simulink model "ackerman_ROS_controller_neuronal"  (R2024a)
settings: Solver=FixedStepDiscrete  StartTime=0.0  StopTime=70  FixedStep=0.1  RelTol=1e-3
undefined symbols (not defined in the file or in its folder): Angular, Linear
libraries: neural x47, robotlib x15, robotcorelib x1
(part 2 of 2)

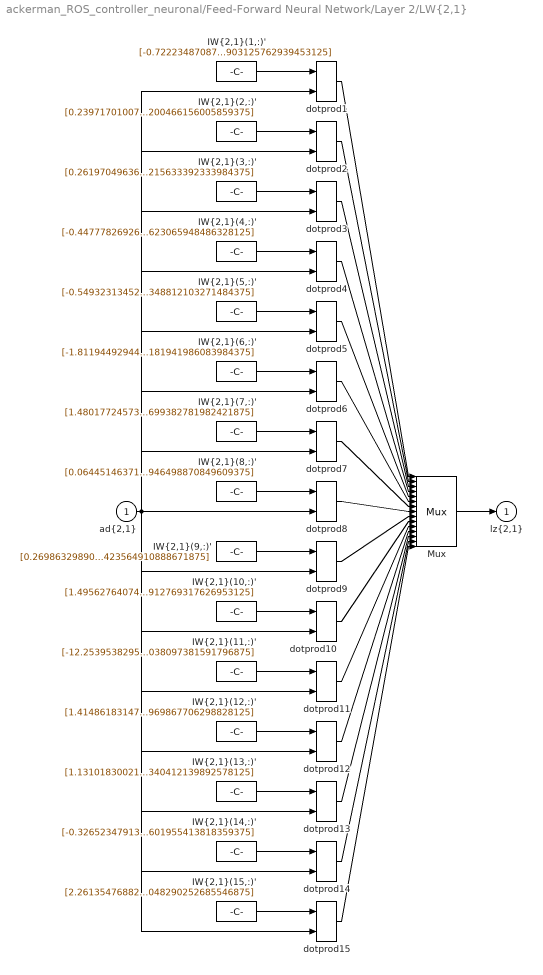
== system ackerman_ROS_controller_neuronal/Feed-Forward Neural Network/Layer 2/LW{2,1} ==
  "ad{2,1}" : Inport  PortDimensions=25  SampleTime=0.1
      mask Display: e = 0.06;c1 = [120 230 180]/255;c2 = ([120 230 180]+0)/(256+128);c3 = ([120 230 180]+128)/(256+128);patch([0 1 1 0],[0 0 1 1],c1);patch([0 1 1 1-e 1-e 0+e],[0 0 1 1-e 0+e 0+e],c2);patch([0 0 1 1-e 0+e 0+e],[0 1 1 1-e 1-e 0+e],c3);plot([0 1 1 0 0],[0 0 1 1 0]);
  "IW{2,1}(1,:)'" : Constant  Value=[-0.7222348708729093846869773187790997326374053955078125;0.0981793588010296536250365306841558776795864105224609375;0.1371759683882359526219119061352103017270565032958984375;0.0730258607750217392240443814444006420671939849853515625;-1.372802742190014857470714559894986450672149658203125;-1.8212743748848574387722010214929468929767608642578125;-1.5267678279169134558657106026657857000827789306640625;1.4479084045406518388432459687464870512485504150390625;-0.13063321599715915777295549560221843421459197998046875;1.712382502643198467495722070452757179737091064453125;-0.1827473613784254269365447953532566316425800323486328125;-1.0574757090524122826735720082069747149944305419921875;-1.0665010937239696175993231008760631084442138671875;-0.9024666040768736241517444796045310795307159423828125;-1.8865157325392905018901501534855924546718597412109375;1.318039630886072899329519714228808879852294921875;1.1464077279038644707753746843081898987293243408203125;-0.97169709672360526919732137685059569776058197021484375;-2.487878129250618020051888379384763538837432861328125;-0.9738457646549019131043678498826920986175537109375;0.34793062286432674401481790482648648321628570556640625;0.01100840170375953601389351632633406552486121654510498046875;1.6560578546683313305720730568282306194305419921875;-2.101274677924584555199771784828044474124908447265625;2.983503581776024038418881900724954903125762939453125]
      mask Display: e = 0.06;c1 = [120 150 230]/255;c2 = ([120 150 230]+0)/383;c3 = ([120 150 230]+128)/383;patch([0 1 1 0],[0 0 1 1],c1);patch([0 1 1 1-e 1-e 0+e],[0 0 1 1-e 0+e 0+e],c2);patch([0 0 1 1-e 0+e 0+e],[0 1 1 1-e 1-e 0+e],c3);plot([0 1 1 0 0],[0 0 1 1 0]);disp('weights');
  "IW{2,1}(10,:)'" : Constant  Value=[1.4956276407477755441277622594498097896575927734375;-0.788962805301818281833448054385371506214141845703125;0.269669087111882144203178768293582834303379058837890625;-0.292657048209959469442509316650102846324443817138671875;-2.133692028425654196865934864035807549953460693359375;-0.39117674700785476371578397447592578828334808349609375;0.581263930568486131278405082412064075469970703125;0.97155478441386866617079931529588066041469573974609375;-2.073983957749963025207762257196009159088134765625;2.731327761950456789463714812882244586944580078125;-0.4915888766656066888316445329110138118267059326171875;-2.3179880946341011593858638661913573741912841796875;0.09301131783168821443030793716388870961964130401611328125;0.1436793922233029208168630930231302045285701751708984375;-1.64205595454593389348474374855868518352508544921875;0.2132037752463056268226182510261423885822296142578125;0.27785129634182259561470118569559417665004730224609375;1.5674675258729935389823140212683938443660736083984375;-0.8311551921900461881165256272652186453342437744140625;-1.7108512116470517838706655311398208141326904296875;0.07415612580187225244543469671043567359447479248046875;-0.55140252940727052521907580739934928715229034423828125;-1.38513208025195666550644091330468654632568359375;0.1518428514926022654396575717328232713043689727783203125;2.596690078219698438743989754584617912769317626953125]
      mask Display: e = 0.06;c1 = [120 150 230]/255;c2 = ([120 150 230]+0)/383;c3 = ([120 150 230]+128)/383;patch([0 1 1 0],[0 0 1 1],c1);patch([0 1 1 1-e 1-e 0+e],[0 0 1 1-e 0+e 0+e],c2);patch([0 0 1 1-e 0+e 0+e],[0 1 1 1-e 1-e 0+e],c3);plot([0 1 1 0 0],[0 0 1 1 0]);disp('weights');
  "IW{2,1}(11,:)'" : Constant  Value=[-12.253953829568370537117516505531966686248779296875;4.39303208527887623091601199121214449405670166015625;0.38223307212810386790380334787187166512012481689453125;-1.9037658357750879556391510050161741673946380615234375;-0.95260750474161459688815511981374584138393402099609375;5.360034857704107480458333157002925872802734375;6.67310871356777823848460684530436992645263671875;2.729141390269420153202872825204394757747650146484375;-1.915432689159779489074253433500416576862335205078125;-1.018409021534567582278896225034259259700775146484375;0.3096668608063126715279622658272273838520050048828125;-0.356772271992063794154859124319045804440975189208984375;-3.5098980230815488567941429209895431995391845703125;-2.42911505781934788927856061491183936595916748046875;-3.80273708191338233319811479304917156696319580078125;2.49722685927970733388292501331306993961334228515625;-0.8878414190837864428118564319447614252567291259765625;2.402914930610447807879381798557005822658538818359375;-0.5057975403114471912857652569073252379894256591796875;7.45380146518667441313255039858631789684295654296875;1.7300526442494590373399887539562769234180450439453125;2.665766658331240268609008126077242195606231689453125;1.8102918202158633231846351918647997081279754638671875;-0.98601708086775996520145781687460839748382568359375;1.442751514700642445632183807902038097381591796875]
      mask Display: e = 0.06;c1 = [120 150 230]/255;c2 = ([120 150 230]+0)/383;c3 = ([120 150 230]+128)/383;patch([0 1 1 0],[0 0 1 1],c1);patch([0 1 1 1-e 1-e 0+e],[0 0 1 1-e 0+e 0+e],c2);patch([0 0 1 1-e 0+e 0+e],[0 1 1 1-e 1-e 0+e],c3);plot([0 1 1 0 0],[0 0 1 1 0]);disp('weights');
  "IW{2,1}(12,:)'" : Constant  Value=[1.414861831478989362409492969163693487644195556640625;1.2707933400524071831938499599345959722995758056640625;1.34394123583657698617344067315571010112762451171875;1.5462306076190726056296398382983170449733734130859375;-5.17509624264692735806647760909982025623321533203125;2.824180089653766767554543548612855374813079833984375;-1.82988593402526600328883432666771113872528076171875;-3.2592273475407065319586763507686555385589599609375;-1.928758399229578923694816694478504359722137451171875;-1.34087555628182286682203994132578372955322265625;-5.07940803163818177523580743581987917423248291015625;1.5511947868706601472155170995392836630344390869140625;-2.096771476592278471429153796634636819362640380859375;0.90357692537882805527971186165814287960529327392578125;-1.337567839827941806873923269449733197689056396484375;-0.79672981490855487862745576421730220317840576171875;-0.4541749841010995769607916372478939592838287353515625;2.14134792906865190076359795057214796543121337890625;-3.362985062282791037802098799147643148899078369140625;-1.466686761802152627609530100016854703426361083984375;-4.816526752401596667141348007135093212127685546875;1.9420442507405712984080992100643925368785858154296875;0.1615625324561887066199261653309804387390613555908203125;-0.04622279232351557409774756024489761330187320709228515625;3.825540516566335202952586769242770969867706298828125]
      mask Display: e = 0.06;c1 = [120 150 230]/255;c2 = ([120 150 230]+0)/383;c3 = ([120 150 230]+128)/383;patch([0 1 1 0],[0 0 1 1],c1);patch([0 1 1 1-e 1-e 0+e],[0 0 1 1-e 0+e 0+e],c2);patch([0 0 1 1-e 0+e 0+e],[0 1 1 1-e 1-e 0+e],c3);plot([0 1 1 0 0],[0 0 1 1 0]);disp('weights');
  "IW{2,1}(13,:)'" : Constant  Value=[1.131018300215737237834900952293537557125091552734375;4.6569848027918627764165648841299116611480712890625;0.2344222257143036836080085549838258884847164154052734375;-1.9242483801722425340585687081329524517059326171875;0.63069029440676704911794558938709087669849395751953125;-0.64797978029724834225788754338282160460948944091796875;1.5346118234120551537813526010722853243350982666015625;-3.07598490301061300300489165238104760646820068359375;-1.0483748074715124598554893964319489896297454833984375;4.582483484907502457872396917082369327545166015625;-0.775742089778314269921111190342344343662261962890625;2.773228499954765169377424172125756740570068359375;-2.9959296210777655034007693757303059101104736328125;-0.93210670025544517525162291349261067807674407958984375;0.57584394096119317918436308900709263980388641357421875;1.672267185378192966282995257643051445484161376953125;1.4951734432408445574225197560735978186130523681640625;-1.1348966277614584985400369987473823130130767822265625;1.0463170313689882373608952548238448798656463623046875;-2.95346669820664242678276423248462378978729248046875;1.6040671880945283067632090023835189640522003173828125;1.7640246337201224147150924181914888322353363037109375;-2.450281737022660166758214472793042659759521484375;0.81620673218923356362353160875500179827213287353515625;-0.003525358734461532528303706612859969027340412139892578125]
      mask Display: e = 0.06;c1 = [120 150 230]/255;c2 = ([120 150 230]+0)/383;c3 = ([120 150 230]+128)/383;patch([0 1 1 0],[0 0 1 1],c1);patch([0 1 1 1-e 1-e 0+e],[0 0 1 1-e 0+e 0+e],c2);patch([0 0 1 1-e 0+e 0+e],[0 1 1 1-e 1-e 0+e],c3);plot([0 1 1 0 0],[0 0 1 1 0]);disp('weights');
  "IW{2,1}(14,:)'" : Constant  Value=[-0.3265234791349171938890094679663889110088348388671875;-1.1396787488998636472814496300998143851757049560546875;0.659566474006498371096540722646750509738922119140625;0.272697770417793972086428766488097608089447021484375;-5.0464894937421629350637886091135442256927490234375;-0.460730509190456605228547459773835726082324981689453125;0.347248761171756681331856952965608797967433929443359375;-1.8789288689546033150890025353874079883098602294921875;-2.372149876109781896360573227866552770137786865234375;-1.47061283460651903709504040307365357875823974609375;0.304297002840665686829169089833158068358898162841796875;0.45927046314568908957909343371284194290637969970703125;0.00965151118650432564283203618060724693350493907928466796875;-0.0089597391306133720989546276314285933040082454681396484375;1.4480728283000530165480768118868581950664520263671875;-0.259619475803844868000425094578531570732593536376953125;-3.23881172172160081146330412593670189380645751953125;1.4267256202362077477374668887932784855365753173828125;0.041194781003231463467617601281745010055601596832275390625;-0.0296330333925509982473389669621610664762556552886962890625;0.143119096384909549879438372954609803855419158935546875;2.041884735769875280908536296919919550418853759765625;-1.60335254904017698862617180566303431987762451171875;0.73699941051827277949115568844717927277088165283203125;0.77850010350764475841600642525008879601955413818359375]
      mask Display: e = 0.06;c1 = [120 150 230]/255;c2 = ([120 150 230]+0)/383;c3 = ([120 150 230]+128)/383;patch([0 1 1 0],[0 0 1 1],c1);patch([0 1 1 1-e 1-e 0+e],[0 0 1 1-e 0+e 0+e],c2);patch([0 0 1 1-e 0+e 0+e],[0 1 1 1-e 1-e 0+e],c3);plot([0 1 1 0 0],[0 0 1 1 0]);disp('weights');
  "IW{2,1}(15,:)'" : Constant  Value=[2.261354768825730499060000511235557496547698974609375;-1.0449084387729128398092370844096876680850982666015625;0.498644497600040315088421039035893045365810394287109375;0.87165995268127527406676335886004380881786346435546875;-0.2117581073043853512327672206083661876618862152099609375;0.589209338323644526980160662787966430187225341796875;0.56663579855300560961239852986182086169719696044921875;-1.712363214106411124504347753827460110187530517578125;-0.21948370763189817278515647558378987014293670654296875;-0.2630627043740132453564228853792883455753326416015625;-0.9383844632776570104937263749889098107814788818359375;0.608847469718369893598719500005245208740234375;-0.84536117835731550140820900196558795869350433349609375;-0.386280090041679902146398717377451248466968536376953125;0.99837546791996378825473357210285030305385589599609375;0.75469207194089904522371625716914422810077667236328125;1.5421940189576950341887595641310326755046844482421875;-1.36341207684782528275491131353192031383514404296875;-0.2430661277789683272221310517124948091804981231689453125;-0.51870593074241233555454755332903005182743072509765625;0.73854121379737935892961786521482281386852264404296875;-1.1794436948531548114971201357548125088214874267578125;0.27331330562690603347419937563245184719562530517578125;-0.3090746830244601728310271937516517937183380126953125;0.6425613674276131614959695070865564048290252685546875]
      mask Display: e = 0.06;c1 = [120 150 230]/255;c2 = ([120 150 230]+0)/383;c3 = ([120 150 230]+128)/383;patch([0 1 1 0],[0 0 1 1],c1);patch([0 1 1 1-e 1-e 0+e],[0 0 1 1-e 0+e 0+e],c2);patch([0 0 1 1-e 0+e 0+e],[0 1 1 1-e 1-e 0+e],c3);plot([0 1 1 0 0],[0 0 1 1 0]);disp('weights');
  "IW{2,1}(2,:)'" : Constant  Value=[0.2397170100764628164480285477111465297639369964599609375;-1.7860235372168258294323095469735562801361083984375;-0.1909341104956231160993951334603480063378810882568359375;1.089794091494230343641902436502277851104736328125;-0.25454316182217018305067313121980987489223480224609375;0.4322605672483723626697837971732951700687408447265625;-0.2048728567615103468568804601090960204601287841796875;1.0010713515385096794574337764061056077480316162109375;0.295535753540752732515528578005614690482616424560546875;1.92087198018925864317907326039858162403106689453125;-1.605335300954486843494350978289730846881866455078125;-0.348238180518220807879714584487373940646648406982421875;-0.213920007137737899771678939941921271383762359619140625;-0.15827597510949320547268825976061634719371795654296875;-1.87095494522964767014627796015702188014984130859375;0.5537583126068204020242546903318725526332855224609375;3.393669821761664540105130072333849966526031494140625;-0.93735669682763977927919540888979099690914154052734375;-0.489971756418236259467136051171110011637210845947265625;-0.52340342207687695630369262289605103433132171630859375;-0.045709986400645892523630919868082855828106403350830078125;-1.6593880364962318996191470432677306234836578369140625;0.298272634381946233350646480175782926380634307861328125;-2.248105500618230667697616809164173901081085205078125;-0.6680062031411961864790782783529721200466156005859375]
      mask Display: e = 0.06;c1 = [120 150 230]/255;c2 = ([120 150 230]+0)/383;c3 = ([120 150 230]+128)/383;patch([0 1 1 0],[0 0 1 1],c1);patch([0 1 1 1-e 1-e 0+e],[0 0 1 1-e 0+e 0+e],c2);patch([0 0 1 1-e 0+e 0+e],[0 1 1 1-e 1-e 0+e],c3);plot([0 1 1 0 0],[0 0 1 1 0]);disp('weights');
  "IW{2,1}(3,:)'" : Constant  Value=[0.261970496368628624761498713269247673451900482177734375;-0.60739888280470599735139103358960710465908050537109375;0.5564599097384554937661960138939321041107177734375;-0.374375860105218893902900845205294899642467498779296875;-0.78299327263608053950605381032801233232021331787109375;0.06357714215609898411596390133126988075673580169677734375;1.4192641090693587369031547495978884398937225341796875;2.51693998010587183244979314622469246387481689453125;5.6294623510423189571838520350866019725799560546875;-1.286464539985229027507784849149174988269805908203125;-0.12354346668453076996119222030756645835936069488525390625;-1.1111505971322819252833369318977929651737213134765625;0.91159341951149153171485295388265512883663177490234375;-0.39232622808146577764176754499203525483608245849609375;0.1402175853463884236393965920797199942171573638916015625;0.56925765277390716345706778156454674899578094482421875;0.92059763213383638547071541324839927256107330322265625;0.94367513594503582563532972926623187959194183349609375;0.10236138442994859032442178659039200283586978912353515625;-4.77041041420481537471687261131592094898223876953125;0.168770138560168536656647120253182947635650634765625;-0.26194322280417259296569909565732814371585845947265625;-0.475774971764924725636802804729086346924304962158203125;-1.5736736682102014928119615433388389647006988525390625;1.431688367580961962488572680740617215633392333984375]
      mask Display: e = 0.06;c1 = [120 150 230]/255;c2 = ([120 150 230]+0)/383;c3 = ([120 150 230]+128)/383;patch([0 1 1 0],[0 0 1 1],c1);patch([0 1 1 1-e 1-e 0+e],[0 0 1 1-e 0+e 0+e],c2);patch([0 0 1 1-e 0+e 0+e],[0 1 1 1-e 1-e 0+e],c3);plot([0 1 1 0 0],[0 0 1 1 0]);disp('weights');
  "IW{2,1}(4,:)'" : Constant  Value=[-0.44777826926594743728315961561747826635837554931640625;-3.383725423316843006205090205185115337371826171875;-0.78746623535786863801178014909964986145496368408203125;2.1890108502724530126215540803968906402587890625;-0.352996033818494481248961847086320631206035614013671875;-3.3560840870066943608662768383510410785675048828125;-0.47181060041684241834758495315327309072017669677734375;0.1349511593528751329795767333052936010062694549560546875;0.19762711076085504036115025883191265165805816650390625;2.0448312559800871923698650789447128772735595703125;0.351244934439365941170052565212245099246501922607421875;-4.7063534150473866901620567659847438335418701171875;-0.467541956344167675130307770814397372305393218994140625;1.149312339418189221618149531423114240169525146484375;-4.802232561185082460042394814081490039825439453125;-0.86280849768037015667943023800035007297992706298828125;-1.79669457532872645089128127438016235828399658203125;1.9719066394604662928458083115401677787303924560546875;-0.409838122969578666499046448734588921070098876953125;-0.198989210572557084777400859820772893726825714111328125;0.07149902547644758354916660891831270419061183929443359375;0.07893008712068465271283201900587300769984722137451171875;0.221302962972630690163811095771961845457553863525390625;-0.0073554147619722086426374829670749022625386714935302734375;-0.61424249671900554847780995260109193623065948486328125]
      mask Display: e = 0.06;c1 = [120 150 230]/255;c2 = ([120 150 230]+0)/383;c3 = ([120 150 230]+128)/383;patch([0 1 1 0],[0 0 1 1],c1);patch([0 1 1 1-e 1-e 0+e],[0 0 1 1-e 0+e 0+e],c2);patch([0 0 1 1-e 0+e 0+e],[0 1 1 1-e 1-e 0+e],c3);plot([0 1 1 0 0],[0 0 1 1 0]);disp('weights');
  "IW{2,1}(5,:)'" : Constant  Value=[-0.54932313452935621622685857801116071641445159912109375;1.0910646293434489439988510639523155987262725830078125;-0.550997459572583725417871391982771456241607666015625;0.1440901991300558016018129592339391820132732391357421875;1.079140028794803196632301478530280292034149169921875;0.0393398599148337968500754868728108704090118408203125;-1.42049331825403957196840565302409231662750244140625;-2.46595313683236039281609919271431863307952880859375;-6.11661864873186633673185497173108160495758056640625;1.482546098102724752010317388339899480342864990234375;0.1837285961685906909846011103581986390054225921630859375;1.43912910781371206070389234810136258602142333984375;-0.83114604279066173209145063083269633352756500244140625;0.3330890344646586509469443626585416495800018310546875;0.1023900423496056644179219574652961455285549163818359375;-0.41490769304872487932556168743758462369441986083984375;-1.67760295446157581267243585898540914058685302734375;-1.06127431917100611968862722278572618961334228515625;-0.003065978537111575287499309894201360293664038181304931640625;4.34655159502920351854982072836719453334808349609375;-0.1534842309716845931699680249948869459331035614013671875;0.400954992105880148045571331749670207500457763671875;-0.1424249249246918314071308486745692789554595947265625;1.792772894424814467129181139171123504638671875;-1.5467757263475065965252497335313819348812103271484375]
      mask Display: e = 0.06;c1 = [120 150 230]/255;c2 = ([120 150 230]+0)/383;c3 = ([120 150 230]+128)/383;patch([0 1 1 0],[0 0 1 1],c1);patch([0 1 1 1-e 1-e 0+e],[0 0 1 1-e 0+e 0+e],c2);patch([0 0 1 1-e 0+e 0+e],[0 1 1 1-e 1-e 0+e],c3);plot([0 1 1 0 0],[0 0 1 1 0]);disp('weights');
  "IW{2,1}(6,:)'" : Constant  Value=[-1.8119449294403484618243282966432161629199981689453125;2.444318837039485714512920822016894817352294921875;-0.07368112505512285081987755575028131715953350067138671875;-2.145700779201991093003698551910929381847381591796875;-0.9572739438411834722586490897811017930507659912109375;-0.188121891721915679429599776995019055902957916259765625;0.9611308056030114510548401085543446242809295654296875;2.94159370729522873233463542419485747814178466796875;0.72461548946288811823279729651403613388538360595703125;7.4813950876740147322152552078478038311004638671875;-0.697399432913040850934294212493114173412322998046875;5.19645893463261199229918929631821811199188232421875;-2.741024559107590352624583829310722649097442626953125;-0.97255815270820733520196199606289155781269073486328125;-1.2445654616562291661097106043598614633083343505859375;7.672483445518057720846627489663660526275634765625;-3.078001255765624222249243757687509059906005859375;2.84873546773435837309307316900230944156646728515625;-1.4631297617049445758397041572607122361660003662109375;2.49430001537067891348442572052590548992156982421875;0.461656941310882251716662949547753669321537017822265625;-1.9419212872258782009993183237384073436260223388671875;4.79264735456007873182215917040593922138214111328125;1.882245256892961293715416104532778263092041015625;-1.0480916894411025364064471432357095181941986083984375]
      mask Display: e = 0.06;c1 = [120 150 230]/255;c2 = ([120 150 230]+0)/383;c3 = ([120 150 230]+128)/383;patch([0 1 1 0],[0 0 1 1],c1);patch([0 1 1 1-e 1-e 0+e],[0 0 1 1-e 0+e 0+e],c2);patch([0 0 1 1-e 0+e 0+e],[0 1 1 1-e 1-e 0+e],c3);plot([0 1 1 0 0],[0 0 1 1 0]);disp('weights');
  "IW{2,1}(7,:)'" : Constant  Value=[1.4801772457355346634955139961675740778446197509765625;1.318711367776444820520964640309102833271026611328125;0.30247197048828600163261626221355982124805450439453125;0.61158145662743967907459818889037705957889556884765625;7.04417940959445498805280294618569314479827880859375;2.813147376453120074302205466665327548980712890625;2.02823398638439922336829113191924989223480224609375;4.49407814670192440331675243214704096317291259765625;1.0110350640216620998756980043253861367702484130859375;1.2801997511761538106611624243669211864471435546875;-2.12176970852421309388091685832478106021881103515625;1.04524485829133784164923781645484268665313720703125;0.3049728969043636883640147061669267714023590087890625;0.0087954731394813100153751150855896412394940853118896484375;2.037032988746230177667939642560668289661407470703125;-0.66488674366804279003417832427658140659332275390625;4.90415931461289034132278175093233585357666015625;-1.8438657142552286050118937055231072008609771728515625;-1.38936982711239576104844672954641282558441162109375;0.1668950879160215061691729943049722351133823394775390625;-0.232769268003413076773000511821010150015354156494140625;-1.4889464777319803001631726147024892270565032958984375;2.04632617167272901070873558637686073780059814453125;5.3200910569059036703265519463457167148590087890625;3.717293199985980844957111912663094699382781982421875]
      mask Display: e = 0.06;c1 = [120 150 230]/255;c2 = ([120 150 230]+0)/383;c3 = ([120 150 230]+128)/383;patch([0 1 1 0],[0 0 1 1],c1);patch([0 1 1 1-e 1-e 0+e],[0 0 1 1-e 0+e 0+e],c2);patch([0 0 1 1-e 0+e 0+e],[0 1 1 1-e 1-e 0+e],c3);plot([0 1 1 0 0],[0 0 1 1 0]);disp('weights');
  "IW{2,1}(8,:)'" : Constant  Value=[0.06445146371199104995408646345822489820420742034912109375;-0.044183667313972663226451231821556575596332550048828125;-0.35126032250380545551848854302079416811466217041015625;-0.88197883663572096413219014721107669174671173095703125;-2.238882353710103689792276782100088894367218017578125;-1.8444788827616742654669224066310562193393707275390625;-2.691919241931521877830846278811804950237274169921875;-0.1326525602101664702558991848491132259368896484375;-0.98480343280568849451128699001856148242950439453125;1.9990402746472291095614082223619334399700164794921875;-0.56306716680536339492135766704450361430644989013671875;-0.91734017780722865165188295577536337077617645263671875;-0.248471315230862577205783736644661985337734222412109375;-0.081989872966671761833623577331309206783771514892578125;-3.31723769828868331188687079702503979206085205078125;2.539354068363019134579872115864418447017669677734375;1.323678629148659968706169820507057011127471923828125;-1.741735370432359264469823756371624767780303955078125;-3.50180166901319100958289709524251520633697509765625;-0.77495639328703591619529333911486901342868804931640625;0.4932289963934730625538804815732873976230621337890625;-0.73129018207202334256322728833765722811222076416015625;2.205856700377589962869251394295133650302886962890625;-5.95653778005394318739718073629774153232574462890625;4.57463430768000645088022793061099946498870849609375]
      mask Display: e = 0.06;c1 = [120 150 230]/255;c2 = ([120 150 230]+0)/383;c3 = ([120 150 230]+128)/383;patch([0 1 1 0],[0 0 1 1],c1);patch([0 1 1 1-e 1-e 0+e],[0 0 1 1-e 0+e 0+e],c2);patch([0 0 1 1-e 0+e 0+e],[0 1 1 1-e 1-e 0+e],c3);plot([0 1 1 0 0],[0 0 1 1 0]);disp('weights');
  "IW{2,1}(9,:)'" : Constant  Value=[0.26986329890596982838957273997948504984378814697265625;-0.56538183520648654933893340057693421840667724609375;-0.425175329156997461321765285902074538171291351318359375;-2.401161125518981531712370269815437495708465576171875;-1.368104203267849872105443864711560308933258056640625;1.26933535361061355928313787444494664669036865234375;-1.7135990421625690860452095876098610460758209228515625;1.8951159496616483135511543878237716853618621826171875;0.08682832216681928005908019940761732868850231170654296875;0.6048436198441249356250182245275937020778656005859375;-0.02591140475834195766591250276178470812737941741943359375;0.7761671562904066679067227596533484756946563720703125;0.5681043535016152556949009522213600575923919677734375;0.39054935011953018086927613694570027291774749755859375;0.560583128573572508912548073567450046539306640625;0.51134784361988494527651027965475805103778839111328125;4.650532288156941973511493415571749210357666015625;0.248215679602704797357404231661348603665828704833984375;-0.0820972492757883198777335564955137670040130615234375;-2.472415154133799308766583635588176548480987548828125;-0.460550177661596393807741378623177297413349151611328125;-0.5630392402789017314290731519577093422412872314453125;-4.29550074795379988046306607429869472980499267578125;-0.23483040235492647074266869822167791426181793212890625;2.764285081659891840644149851868860423564910888671875]
      mask Display: e = 0.06;c1 = [120 150 230]/255;c2 = ([120 150 230]+0)/383;c3 = ([120 150 230]+128)/383;patch([0 1 1 0],[0 0 1 1],c1);patch([0 1 1 1-e 1-e 0+e],[0 0 1 1-e 0+e 0+e],c2);patch([0 0 1 1-e 0+e 0+e],[0 1 1 1-e 1-e 0+e],c3);plot([0 1 1 0 0],[0 0 1 1 0]);disp('weights');
  Mux : Mux  Inputs=15
      mask Display: e = 0.06;c1 = [120 150 230]/255;c2 = ([120 150 230]+0)/383;c3 = ([120 150 230]+128)/383;patch([0 1 1 0],[0 0 1 1],c1);patch([0 1 1 1-e 1-e 0+e],[0 0 1 1-e 0+e 0+e],c2);patch([0 0 1 1-e 0+e 0+e],[0 1 1 1-e 1-e 0+e],c3);plot([0 1 1 0 0],[0 0 1 1 0]);disp('Mux');
  dotprod{1..15} (15 alike) : neural/Weight Functions/dotprod
  "lz{2,1}" : Outport
      mask Display: e = 0.06;c1 = [120 230 180]/255;c2 = ([120 230 180]+0)/(256+128);c3 = ([120 230 180]+128)/(256+128);patch([0 1 1 0],[0 0 1 1],c1);patch([0 1 1 1-e 1-e 0+e],[0 0 1 1-e 0+e 0+e],c2);patch([0 0 1 1-e 0+e 0+e],[0 1 1 1-e 1-e 0+e],c3);plot([0 1 1 0 0],[0 0 1 1 0]);
  wires:
  "IW{2,1}(1,:)'"/1 -> dotprod1/1
  "ad{2,1}"/1 -> dotprod1/2, dotprod2/2, dotprod3/2, dotprod4/2, dotprod5/2, dotprod6/2, dotprod7/2, dotprod8/2, dotprod9/2, dotprod10/2, dotprod11/2, dotprod12/2, dotprod13/2, dotprod14/2, dotprod15/2
  dotprod1/1 -> Mux/1
  "IW{2,1}(2,:)'"/1 -> dotprod2/1
  dotprod2/1 -> Mux/2
  "IW{2,1}(3,:)'"/1 -> dotprod3/1
  dotprod3/1 -> Mux/3
  "IW{2,1}(4,:)'"/1 -> dotprod4/1
  dotprod4/1 -> Mux/4
  "IW{2,1}(5,:)'"/1 -> dotprod5/1
  dotprod5/1 -> Mux/5
  "IW{2,1}(6,:)'"/1 -> dotprod6/1
  dotprod6/1 -> Mux/6
  "IW{2,1}(7,:)'"/1 -> dotprod7/1
  dotprod7/1 -> Mux/7
  "IW{2,1}(8,:)'"/1 -> dotprod8/1
  dotprod8/1 -> Mux/8
  "IW{2,1}(9,:)'"/1 -> dotprod9/1
  dotprod9/1 -> Mux/9
  "IW{2,1}(10,:)'"/1 -> dotprod10/1
  dotprod10/1 -> Mux/10
  "IW{2,1}(11,:)'"/1 -> dotprod11/1
  dotprod11/1 -> Mux/11
  "IW{2,1}(12,:)'"/1 -> dotprod12/1
  dotprod12/1 -> Mux/12
  "IW{2,1}(13,:)'"/1 -> dotprod13/1
  dotprod13/1 -> Mux/13
  "IW{2,1}(14,:)'"/1 -> dotprod14/1
  dotprod14/1 -> Mux/14
  "IW{2,1}(15,:)'"/1 -> dotprod15/1
  dotprod15/1 -> Mux/15
  Mux/1 -> "lz{2,1}"/1

== system ackerman_ROS_controller_neuronal/Feed-Forward Neural Network/Layer 3/Delays 1 ==
  "p{3}" : Inport  PortDimensions=15  SampleTime=0.1
      mask Display: e = 0.06;c1 = [120 230 180]/255;c2 = ([120 230 180]+0)/(256+128);c3 = ([120 230 180]+128)/(256+128);patch([0 1 1 0],[0 0 1 1],c1);patch([0 1 1 1-e 1-e 0+e],[0 0 1 1-e 0+e 0+e],c2);patch([0 0 1 1-e 0+e 0+e],[0 1 1 1-e 1-e 0+e],c3);plot([0 1 1 0 0],[0 0 1 1 0]);
  mux : Mux  Inputs=1
      mask Display: e = 0.06;c1 = [120 150 230]/255;c2 = ([120 150 230]+0)/383;c3 = ([120 150 230]+128)/383;patch([0 1 1 0],[0 0 1 1],c1);patch([0 1 1 1-e 1-e 0+e],[0 0 1 1-e 0+e 0+e],c2);patch([0 0 1 1-e 0+e 0+e],[0 1 1 1-e 1-e 0+e],c3);plot([0 1 1 0 0],[0 0 1 1 0]);disp('Mux')
  "pd{3,2}" : Outport
      mask Display: e = 0.06;c1 = [120 230 180]/255;c2 = ([120 230 180]+0)/(256+128);c3 = ([120 230 180]+128)/(256+128);patch([0 1 1 0],[0 0 1 1],c1);patch([0 1 1 1-e 1-e 0+e],[0 0 1 1-e 0+e 0+e],c2);patch([0 0 1 1-e 0+e 0+e],[0 1 1 1-e 1-e 0+e],c3);plot([0 1 1 0 0],[0 0 1 1 0]);
  wires:
  "p{3}"/1 -> mux/1
  mux/1 -> "pd{3,2}"/1

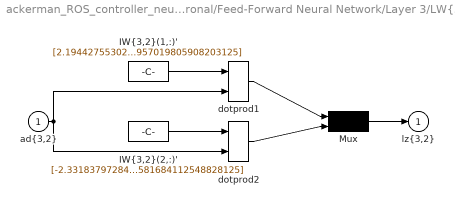
== system ackerman_ROS_controller_neuronal/Feed-Forward Neural Network/Layer 3/LW{3,2} ==
  "ad{3,2}" : Inport  PortDimensions=15  SampleTime=0.1
      mask Display: e = 0.06;c1 = [120 230 180]/255;c2 = ([120 230 180]+0)/(256+128);c3 = ([120 230 180]+128)/(256+128);patch([0 1 1 0],[0 0 1 1],c1);patch([0 1 1 1-e 1-e 0+e],[0 0 1 1-e 0+e 0+e],c2);patch([0 0 1 1-e 0+e 0+e],[0 1 1 1-e 1-e 0+e],c3);plot([0 1 1 0 0],[0 0 1 1 0]);
  "IW{3,2}(1,:)'" : Constant  Value=[2.194427553020759535939987472374923527240753173828125;-2.89315324247352290143453501514159142971038818359375;2.995896655612863224149577945354394614696502685546875;1.0568450907404265404210264023276977241039276123046875;3.07264854392400454941025600419379770755767822265625;0.059963042196349659873622073291699052788317203521728515625;0.685412386988343502736142909270711243152618408203125;-1.4543402617935754506106604821979999542236328125;-3.053787651896501476045386880286969244480133056640625;1.193903030755177230304298063856549561023712158203125;0.371471141146440364533276579095399938523769378662109375;-1.1143526895599877857279125237255357205867767333984375;-1.38901495342764125240364592173136770725250244140625;-1.8811867973388085584218742951634339988231658935546875;3.125063688610009382529142385465092957019805908203125]
      mask Display: e = 0.06;c1 = [120 150 230]/255;c2 = ([120 150 230]+0)/383;c3 = ([120 150 230]+128)/383;patch([0 1 1 0],[0 0 1 1],c1);patch([0 1 1 1-e 1-e 0+e],[0 0 1 1-e 0+e 0+e],c2);patch([0 0 1 1-e 0+e 0+e],[0 1 1 1-e 1-e 0+e],c3);plot([0 1 1 0 0],[0 0 1 1 0]);disp('weights');
  "IW{3,2}(2,:)'" : Constant  Value=[-2.331837972841395600909208951634354889392852783203125;1.951611558838723059494668632396496832370758056640625;-2.9043657663301392091170782805420458316802978515625;-0.80092620706572947852919241995550692081451416015625;-2.994580256764732606455936547718010842800140380859375;-0.1129210205827529123201458105540950782597064971923828125;-0.78526796977570401114832066014059819281101226806640625;1.4520119481208479950140599612495861947536468505859375;2.40869951030250462054027593694627285003662109375;-1.001037494482996503819549616309814155101776123046875;-0.05212098430401361504049617678901995532214641571044921875;4.02695432795678254223048497806303203105926513671875;0.54835649810448428009834742624661885201930999755859375;1.0339056551467449285297561800689436495304107666015625;-1.3952382999627801485331701769609935581684112548828125]
      mask Display: e = 0.06;c1 = [120 150 230]/255;c2 = ([120 150 230]+0)/383;c3 = ([120 150 230]+128)/383;patch([0 1 1 0],[0 0 1 1],c1);patch([0 1 1 1-e 1-e 0+e],[0 0 1 1-e 0+e 0+e],c2);patch([0 0 1 1-e 0+e 0+e],[0 1 1 1-e 1-e 0+e],c3);plot([0 1 1 0 0],[0 0 1 1 0]);disp('weights');
  Mux : Mux  Inputs=2
      mask Display: e = 0.06;c1 = [120 150 230]/255;c2 = ([120 150 230]+0)/383;c3 = ([120 150 230]+128)/383;patch([0 1 1 0],[0 0 1 1],c1);patch([0 1 1 1-e 1-e 0+e],[0 0 1 1-e 0+e 0+e],c2);patch([0 0 1 1-e 0+e 0+e],[0 1 1 1-e 1-e 0+e],c3);plot([0 1 1 0 0],[0 0 1 1 0]);disp('Mux');
  dotprod1 : neural/Weight Functions/dotprod
  dotprod2 : neural/Weight Functions/dotprod
  "lz{3,2}" : Outport
      mask Display: e = 0.06;c1 = [120 230 180]/255;c2 = ([120 230 180]+0)/(256+128);c3 = ([120 230 180]+128)/(256+128);patch([0 1 1 0],[0 0 1 1],c1);patch([0 1 1 1-e 1-e 0+e],[0 0 1 1-e 0+e 0+e],c2);patch([0 0 1 1-e 0+e 0+e],[0 1 1 1-e 1-e 0+e],c3);plot([0 1 1 0 0],[0 0 1 1 0]);
  wires:
  "IW{3,2}(1,:)'"/1 -> dotprod1/1
  "ad{3,2}"/1 -> dotprod1/2, dotprod2/2
  dotprod1/1 -> Mux/1
  "IW{3,2}(2,:)'"/1 -> dotprod2/1
  dotprod2/1 -> Mux/2
  Mux/1 -> "lz{3,2}"/1

== matlab function ackerman_ROS_controller_neuronal/ROS Robot/Conversion_diff_ackerman ==
  data: steering_wheel_angle input; V output; linear_vel_ackerman_kmh input; W output
function [V,W] = fcn(steering_wheel_angle, linear_vel_ackerman_kmh)

    %Aproximacion de angulo volante y velocidad linal a vel_linar y angular.
    % *************************************
    
    min_turning_radius_vehicle = 2;  % radio de giro del vehiculo. Radio minimo en el que gira 180 grados. 
    max_turning_radius_vehicle = 34; % radio de giro del vehiculo. Radio máximo con el volante girado 1º
    max_steering_wheel_angle = 90;  % angulo máximo de volante permitido (grados).
    max_vehicle_linear_speed = 50;  % velocidad máxima de vehiculo (km/h).
    
    
    % Filtrado des los valores máximos
    
    if steering_wheel_angle > max_steering_wheel_angle
        steering_wheel_angle = max_steering_wheel_angle;  
    end
    
    if steering_wheel_angle < (-1*max_steering_wheel_angle)
        steering_wheel_angle = max_steering_wheel_angle;  
    end
    
    if linear_vel_ackerman_kmh > max_vehicle_linear_speed
        linear_vel_ackerman_kmh = max_vehicle_linear_speed;
    end
    
    
    %Conversion a m/s
    linear_vel_ackerman_ms = linear_vel_ackerman_kmh/3.6; %(m/s)
    
    %Conversion a linear and angular velocity for the simulator.
    % v=rω --> ω = v/r
    
    % max_steering_wheel_angle -- > min_turning_radius_vehicle
    % steering_wheel_angle = 0 --> angular_vel_vehicle = 0;
    
    turning_radius = (max_turning_radius_vehicle-((max_turning_radius_vehicle-min_turning_radius_vehicle)/max_steering_wheel_angle)*abs(steering_wheel_angle));
    
    if steering_wheel_angle > 0
            turning_radius = turning_radius;
    elseif steering_wheel_angle < 0
            turning_radius = -1*turning_radius;
    end
    
    if abs(steering_wheel_angle) < 0.01
        angular_vel_vehicle = 0;
    else
        angular_vel_vehicle = linear_vel_ackerman_ms / turning_radius;
    end
    
    %Sin velocidad linear, tampoco debe girar
    
    if linear_vel_ackerman_ms == 0
        angular_vel_vehicle = 0;
    end
    
    
    %Rellenamos los campos del mensaje V y W
    V= linear_vel_ackerman_ms;

    W=angular_vel_vehicle;
    
    
    %********************************************************

== matlab function ackerman_ROS_controller_neuronal/ROS Robot/MATLAB Function ==
  data: u input; y output
function y = fcn(u)
u(isinf(u))=15.0;
y = u;

== matlab function ackerman_ROS_controller_neuronal/MATLAB Function ==
  data: stop_flag input; vel output; vel input; steering_wheel input; steering_wheel output
function [vel, steering_wheel]= stop(stop_flag,vel,steering_wheel)
    if stop_flag 
        steering_wheel=0;
        vel=0;
    else
        vel=vel;
        steering_wheel=steering_wheel;
    end

== matlab function ackerman_ROS_controller_neuronal/Evaluacion_maniobra/evaluacion_fin ==
  data: clock input; x input; y input; theta input; stop_flag output
function stop_flag = evaluacion_fin(clock, x, y, theta)
    if x > 59 && x < 60
        if y < 4
            stop_flag = 1;
        else 
            stop_flag = 0;
        end
        else
            stop_flag = 0;
    end
end
